simulink subsystem "Fixed_Restriction_With_Cavitation"  (R2020b)
settings: Solver=VariableStepAuto  StartTime=0.0  StopTime=10.0  RelTol=1e-3
model mask{Cv=0.5, x_T=0.3}
  mask prompts: Cv "Cv Flow Coefficient (Imperial Units)"; x_T "x_T Threshold Choked Pressure Drop Ratio Factor for compressible gas flow calculation (=dP_Choked/P1)"
libraries: nesl_utility x2, SimscapeCustomBlocks_lib x1
settings Model: Creator=Edward  LastModifiedBy=Edward

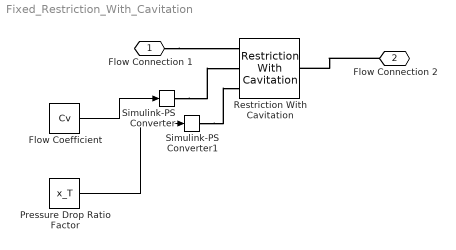
== system Fixed_Restriction_With_Cavitation ==
  Flow Coefficient : Constant  Value=Cv
  Pressure Drop Ratio Factor : Constant  Value=x_T
  Restriction With Cavitation : SimscapeCustomBlocks_lib/Restriction With Cavitation  area=2e-5 m^2  F_L=0.45  F_d=1  X_liquid_threshold=0.6  X_gas_theshold=0.9
      settings: InternalSimscapePortConfiguration="{\"Bottom\":[],\"Left\":[{\"id\":\"A\",\"label\":\"A\",\"type\":\"foundation.two_phase_fluid.two_phase_fluid\"},{\"id\":\"Cv\",\"label\":\"Cv\",\"type\":\"input\"},{\"id\":\"x_T\",\"label\":\"x_T\",\"type\":\"input\"}],\"Right\":[{\"id\":\"B\",\"label\":\"B\",\"type\":\"foundation.two_phase_fluid.two_phase_fluid\"}],\"Top\":[]}"
  Simulink-PS Converter : nesl_utility/Simulink-PS Converter  PhysicalDomain=network_engine_domain  SubClassName=ps_input  LeftPortType=input  RightPortType=output  PseudoPeriodic=off  Frequencies=[]  NoiseDistribution=none  NoiseParameters=[]  Unit=1  AffineConversion=off  FilteringAndDerivatives=provide  SimscapeFilterOrder=1  InputFilterTimeConstant=0.001  UdotUserProvided=0
  Simulink-PS Converter1 : nesl_utility/Simulink-PS Converter  PhysicalDomain=network_engine_domain  SubClassName=ps_input  LeftPortType=input  RightPortType=output  PseudoPeriodic=off  Frequencies=[]  NoiseDistribution=none  NoiseParameters=[]  Unit=1  AffineConversion=off  FilteringAndDerivatives=provide  SimscapeFilterOrder=1  InputFilterTimeConstant=0.001  UdotUserProvided=0
  Flow Connection 1 : PMIOPort  Side=Left
  Flow Connection 2 : PMIOPort  Port=2  Side=Right
  wires:
  Flow Coefficient/1 -> Simulink-PS Converter/1
  Pressure Drop Ratio Factor/1 -> Simulink-PS Converter1/1
  connections:
  Flow Connection 1/RConn1 -- Restriction With Cavitation/LConn1
  Simulink-PS Converter/RConn1 -- Restriction With Cavitation/LConn2
  Simulink-PS Converter1/RConn1 -- Restriction With Cavitation/LConn3
  Flow Connection 2/RConn1 -- Restriction With Cavitation/RConn1
